simulink model "Test14Dof"  (R2024a)
settings: Solver=ode4  StartTime=0.0  StopTime=10.0  FixedStep=0.001  RelTol=1e-3
values from neighbouring files (symbols this model uses):
  EnvGrvty = 9.81    [Par.m]
  PlntBattChrgMax = 4.493    [Par.m]
  PlntBattNumCellSer = 96    [Par.m]
  PlntBattOpenCirctVolt = [3.17242 3.17242 3.17242 3.17242 3.17242 3.17242 3.17242;3.18272 3.18272 3.18272 3.18272 3.18272 3.18272 3.18272;3.19302 3.19302 3.19302 3.19302 3.19302 3.19302 3.19302;3.20331 3.20331 3.20331 3.20331 3.20331 3.20331 3.20331;3.21361 3.21361 3.21361 3.21361 3.21361 3.21361 3.21361;3.22391 3.22391 3.22391 3.22391 3.22391 3.22391 3.22391;3.23421 3.23421 3.23421 3.23421 3.23421 3.23421 3.23421;3.24451 ...(+5187 chars)    [Par.m]
  PlntBattSocInit = 0.6    [Par.m]
  PlntBattTempBpt = [-40 -30 -20 0 23 45 60]    [Par.m]
  PlntBattTempInitDegC = 25    [Par.m]
  PlntBattVoltSocBpt = [0 0.01 0.02 0.03 0.04 0.05 0.06 0.07 0.08 0.09 0.1 0.11 0.12 0.13 0.14 0.15 0.16 0.17 0.18 0.19 0.2 0.21 0.22 0.23 0.24 0.25 0.26 0.27 0.28 0.29 0.3 0.31 0.32 0.33 0.34 0.35 0.36 0.37 0.38 0.39 0.4 0.41 0.42 0.43 0.44 0.45 0.46 0.47 0.48 0.49 0.5 0.51 0.52 0.53 0.54 0.55 0.56 0.57 0.58 0.59 0.6 0.61 0.62 0.63 0.64 0.65 0.66 0.67 0.68 0.69 0.7 0.71 0.72 0.73 0.74 0.75 0.76 0.77 0.78 0.79 0.8 0.81  ...(+91 chars)    [Par.m]
  PlntDCDCVoltInit = 650    [Par.m]
  PlntDriveshftDamp = 100    [Par.m]
  PlntDriveshftStiff = 500    [Par.m]
  PlntEM1RotDamp = 0.001    [Par.m]
  PlntEM1RotInertia = 0.01    [Par.m]
  PlntEM2RotDamp = 0.001    [Par.m]
  PlntEM2RotInertia = 0.01    [Par.m]
  PlntEM3RotDamp = 0.001    [Par.m]
  PlntEM3RotInertia = 0.01    [Par.m]
  PlntEM4RotDamp = 0.001    [Par.m]
  PlntEM4RotInertia = 0.01    [Par.m]
  PlntEMWhlGearRatioFL = 11.04    [Par.m]
  PlntEMWhlGearRatioFR = 11.04    [Par.m]
  PlntEMWhlGearRatioRL = 11.04    [Par.m]
  PlntEMWhlGearRatioRR = 11.04    [Par.m]
  PlntSteerGearRatio = 52.025    [Par.m]
  PlntVehCGHgtAxl = 0.375    [Par.m]
  PlntVehDstCGFrntAxl = 1.61    [Par.m]
  PlntVehDstCGRearAxl = 1.39    [Par.m]
  PlntVehFrntUnsprgMass = 100    [Par.m]
  PlntVehInitLatPos = 0    [Par.m]
  PlntVehInitLatVel = 0    [Par.m]
  PlntVehInitLongPos = 0    [Par.m]
  PlntVehInitLongVel = 0    [Par.m]
  PlntVehInitPitchAng = 0    [Par.m]
  PlntVehInitPitchRate = 0    [Par.m]
  PlntVehInitRollAng = 0    [Par.m]
  PlntVehInitRollRate = 0    [Par.m]
  PlntVehInitVertPos = 0    [Par.m]
  PlntVehInitVertVel = 0    [Par.m]
  PlntVehInitYawAng = 0    [Par.m]
  PlntVehInitYawRate = 0    [Par.m]
  PlntVehMass = 2497    [Par.m]
  PlntVehPitchMomentInertia = 1922.7    [Par.m]
  PlntVehRearUnsprgMass = 100    [Par.m]
  PlntVehRollMomentInertia = 432.33333333333331    (= 432.333333333)    [Par.m]
  PlntVehTrckWdth = [1.685,1.685]    [Par.m]
  PlntVehYawMomentInertia = 2066    [Par.m]
  PlntWhlNumFrnt = 2    [Par.m]
  PlntWhlNumRear = 2    [Par.m]
  PlntWhlPrsFrnt = 220000    [Par.m]
  PlntWhlPrsRear = 220000    [Par.m]
undefined symbols (not defined in the file or in its folder): BdyFrm, InertFrm, PlntTrnsfrCaseAxlSpdLock, PlntTrnsfrCaseTrqSplitRatio
libraries: autolibsharedcoupling x12, autolibsharedcommon x12, autolibutils x10, autolibmappedmotor x4, autolibcoupling x4, matrix_library x4, vehdynlibsuspension x2, vehdynlibtire x2, vehdynlibtirecommon x2, vehdynlibsteering x2, shared6dof x2, autolibdatasheetbattery x1
(part 4 of 7)

== system Test14Dof/Subsystem/Vehicle 14 DoF model/Front Suspension/Wheel2SuspFrntOnly ==
  Veh : Inport
  Wheels : Inport  Port=2
  SuspWheel : Inport  Port=3
  Bus Creator : BusCreator  Inputs=2
  Bus Creator1 : BusCreator  Inputs=2
  Bus Selector : BusSelector  OutputSignals=Fext,WhlAng
  Bus Selector7 : BusSelector  OutputSignals=Omega,Fx,Fy,Mx,My,Mz,Re,z,zdot,Kappa,Alpha
  Constant : Constant  Value=repmat(eye(3),[1,1,PlntWhlNumFrnt])
  Math Function : Math  Operator=transpose  SignedPower=on
  Math Function1 : Math  Operator=transpose  SignedPower=on
  Reshape3 : Reshape
  Reshape4 : Reshape
  Selector2 : Selector  NumberOfDimensions=2  InputPortWidth=3  IndexOptions=Index vector (dialog),Select all  Indices=3,1  OutputSizes=1,1
  Selector3 : Selector  NumberOfDimensions=2  InputPortWidth=3  IndexOptions=Index vector (dialog),Select all  Indices=1,1  OutputSizes=1,1
  Signal Specification : SignalSpecification  Dimensions=PlntWhlNumFrnt
  Signal Specification1 : SignalSpecification  Dimensions=PlntWhlNumFrnt
  Signal Specification2 : SignalSpecification  Dimensions=PlntWhlNumFrnt
  Suspension Routing : Subsystem
  Vector Concatenate1 : Concatenate  NumInputs=3  Mode=Multidimensional array  ConcatenateDimension=2
  Vector Concatenate8 : Concatenate  NumInputs=3  Mode=Multidimensional array  ConcatenateDimension=2
  Wheel to Body Transform : Subsystem
  Wheels2Susp : Outport  VectorParamsAs1DForOutWhenUnconnected=off
  wires:
  Signal Specification1/1 -> Vector Concatenate8/2
  Signal Specification/1 -> Vector Concatenate8/1
  Veh/1 -> Suspension Routing/13(Veh)
  Bus Creator/1 -> Bus Creator1/2  "Steering"
  Reshape3/1 -> Bus Creator/2  "WhlCmb"
  Suspension Routing/1(SuspFrame) -> Bus Creator1/1  "SuspFrame"
  Bus Creator1/1 -> Wheels2Susp/1
  Reshape4/1 -> Bus Creator/1  "WhlAng"
  Wheel to Body Transform/3(Fz) -> Suspension Routing/4(Fz)  "Fz"
  Bus Selector/2 -> [WheelAngles], Wheel to Body Transform/4(WheelAngles)  "<WhlAng>"
  Wheels/1 -> Bus Selector7/1
  Math Function/1 -> Wheel to Body Transform/1(Forces)
  Vector Concatenate8/1 -> Math Function/1
  Wheel to Body Transform/1(Fx) -> Suspension Routing/2(Fx)  "Fx"
  Wheel to Body Transform/2(Fy) -> Suspension Routing/3(Fy)  "Fy"
  SuspWheel/1 -> Bus Selector/1
  Bus Selector/1 -> Signal Specification2/1  "<Fext>"
  Signal Specification2/1 -> Vector Concatenate8/3
  Selector2/1 -> Reshape4/1
  [WheelAngles] -> Selector2/1, Selector3/1
  Selector3/1 -> Reshape3/1
  Wheel to Body Transform/4(Mx) -> Suspension Routing/5(<Mx>)
  Wheel to Body Transform/5(My) -> Suspension Routing/6(<My>)
  Wheel to Body Transform/6(Mz) -> Suspension Routing/7(<Mz>)
  Vector Concatenate1/1 -> Math Function1/1
  Math Function1/1 -> Wheel to Body Transform/2(Moments)
  Constant/1 -> Wheel to Body Transform/3(DCM)
  Bus Selector7/1 -> Suspension Routing/1(Omega)  "<Omega>"
  Bus Selector7/2 -> Signal Specification/1  "<Fx>"
  Bus Selector7/3 -> Signal Specification1/1  "<Fy>"
  Bus Selector7/4 -> Vector Concatenate1/1  "<Mx>"
  Bus Selector7/5 -> Vector Concatenate1/2  "<My>"
  Bus Selector7/6 -> Vector Concatenate1/3  "<Mz>"
  Bus Selector7/7 -> Wheel to Body Transform/5(Re), Suspension Routing/8(<Re>)  "<Re>"
  Bus Selector7/8 -> Suspension Routing/9(<z>)  "<z>"
  Bus Selector7/9 -> Suspension Routing/10(<zdot>)  "<zdot>"
  Bus Selector7/10 -> Suspension Routing/11(<Kappa>)  "<Kappa>"
  Bus Selector7/11 -> Suspension Routing/12(<Alpha>)  "<Alpha>"

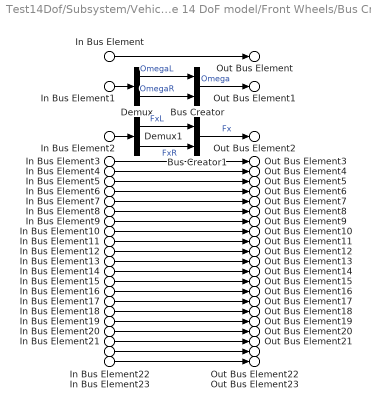
== system Test14Dof/Subsystem/Vehicle 14 DoF model/Front Wheels/Bus Creator ==
  In Bus Element : Inport  PortName=Info  Element=AxlTrq
  In Bus Element1 : Inport  PortName=Info  Element=Omega
  In Bus Element2 : Inport  PortName=Info  Element=Fx
  In Bus Element3 : Inport  PortName=Info  Element=Fy
  In Bus Element4 : Inport  PortName=Info  Element=Fz
  In Bus Element5 : Inport  PortName=Info  Element=Mx
  In Bus Element6 : Inport  PortName=Info  Element=My
  In Bus Element7 : Inport  PortName=Info  Element=Mz
  In Bus Element8 : Inport  PortName=Info  Element=Vx
  In Bus Element9 : Inport  PortName=Info  Element=Vy
  In Bus Element10 : Inport  PortName=Info  Element=Re
  In Bus Element11 : Inport  PortName=Info  Element=Kappa
  In Bus Element12 : Inport  PortName=Info  Element=Alpha
  In Bus Element13 : Inport  PortName=Info  Element=a
  In Bus Element14 : Inport  PortName=Info  Element=b
  In Bus Element15 : Inport  PortName=Info  Element=Gamma
  In Bus Element16 : Inport  PortName=Info  Element=psidot
  In Bus Element17 : Inport  PortName=Info  Element=BrkTrq
  In Bus Element18 : Inport  PortName=Info  Element=BrkPrs
  In Bus Element19 : Inport  PortName=Info  Element=z
  In Bus Element20 : Inport  PortName=Info  Element=zdot
  In Bus Element21 : Inport  PortName=Info  Element=Gnd
  In Bus Element22 : Inport  PortName=Info  Element=GndFz
  In Bus Element23 : Inport  PortName=Info  Element=Prs
  Bus Creator : BusCreator  Inputs=2
  Bus Creator1 : BusCreator  Inputs=2
  Demux : Demux  Outputs=2
  Demux1 : Demux  Outputs=2
  Out Bus Element : Outport  PortName=Wheels  Element=AxlTrq
  Out Bus Element1 : Outport  PortName=Wheels  Element=Omega
  Out Bus Element2 : Outport  PortName=Wheels  Element=Fx
  Out Bus Element3 : Outport  PortName=Wheels  Element=Fy
  Out Bus Element4 : Outport  PortName=Wheels  Element=Fz
  Out Bus Element5 : Outport  PortName=Wheels  Element=Mx
  Out Bus Element6 : Outport  PortName=Wheels  Element=My
  Out Bus Element7 : Outport  PortName=Wheels  Element=Mz
  Out Bus Element8 : Outport  PortName=Wheels  Element=Vx
  Out Bus Element9 : Outport  PortName=Wheels  Element=Vy
  Out Bus Element10 : Outport  PortName=Wheels  Element=Re
  Out Bus Element11 : Outport  PortName=Wheels  Element=Kappa
  Out Bus Element12 : Outport  PortName=Wheels  Element=Alpha
  Out Bus Element13 : Outport  PortName=Wheels  Element=a
  Out Bus Element14 : Outport  PortName=Wheels  Element=b
  Out Bus Element15 : Outport  PortName=Wheels  Element=Gamma
  Out Bus Element16 : Outport  PortName=Wheels  Element=psidot
  Out Bus Element17 : Outport  PortName=Wheels  Element=BrkTrq
  Out Bus Element18 : Outport  PortName=Wheels  Element=BrkPrs
  Out Bus Element19 : Outport  PortName=Wheels  Element=z
  Out Bus Element20 : Outport  PortName=Wheels  Element=zdot
  Out Bus Element21 : Outport  PortName=Wheels  Element=Gnd
  Out Bus Element22 : Outport  PortName=Wheels  Element=GndFz
  Out Bus Element23 : Outport  PortName=Wheels  Element=Prs
  wires:
  In Bus Element16/1 -> Out Bus Element16/1
  In Bus Element10/1 -> Out Bus Element10/1
  In Bus Element3/1 -> Out Bus Element3/1
  In Bus Element18/1 -> Out Bus Element18/1
  In Bus Element12/1 -> Out Bus Element12/1
  In Bus Element11/1 -> Out Bus Element11/1
  In Bus Element20/1 -> Out Bus Element20/1
  In Bus Element13/1 -> Out Bus Element13/1
  In Bus Element8/1 -> Out Bus Element8/1
  In Bus Element14/1 -> Out Bus Element14/1
  In Bus Element15/1 -> Out Bus Element15/1
  In Bus Element17/1 -> Out Bus Element17/1
  In Bus Element19/1 -> Out Bus Element19/1
  In Bus Element22/1 -> Out Bus Element22/1
  In Bus Element21/1 -> Out Bus Element21/1
  In Bus Element23/1 -> Out Bus Element23/1
  In Bus Element1/1 -> Demux/1
  In Bus Element/1 -> Out Bus Element/1
  In Bus Element4/1 -> Out Bus Element4/1
  In Bus Element6/1 -> Out Bus Element6/1
  In Bus Element5/1 -> Out Bus Element5/1
  In Bus Element9/1 -> Out Bus Element9/1
  In Bus Element7/1 -> Out Bus Element7/1
  Demux/1 -> Bus Creator/1  "OmegaL"
  Demux/2 -> Bus Creator/2  "OmegaR"
  Bus Creator/1 -> Out Bus Element1/1  "Omega"
  Bus Creator1/1 -> Out Bus Element2/1  "Fx"
  Demux1/2 -> Bus Creator1/2  "FxR"
  Demux1/1 -> Bus Creator1/1  "FxL"
  In Bus Element2/1 -> Demux1/1

== system Test14Dof/Subsystem/Vehicle 14 DoF model/Front Wheels/Front Friction ==
  u : Inport
  Selector1 : Selector  InputPortWidth=4  IndexOptions=Index vector (dialog)  Indices=[1 2]  OutputSizes=1
  y : Outport
  wires:
  Selector1/1 -> y/1
  u/1 -> Selector1/1

== system Test14Dof/Subsystem/Vehicle 14 DoF model/Front Wheels/Front Ground ==
  u : Inport
  Selector1 : Selector  InputPortWidth=4  IndexOptions=Index vector (dialog)  Indices=[1 2]  OutputSizes=1
  y : Outport
  wires:
  u/1 -> Selector1/1
  Selector1/1 -> y/1

== system Test14Dof/Subsystem/Vehicle 14 DoF model/Front Wheels/MF Tires Vector ==
  BrkPrs : Inport
  AxlTrq : Inport  Port=2
  Vx : Inport  Port=3
  Vy : Inport  Port=4
  Camber : Inport  Port=5
  YawRate : Inport  Port=6
  Fext : Inport  Port=7
  Prs : Inport  Port=8  Unit=Pa
  ScaleFctrs : Inport  Port=9  Unit=1
  Gnd : Inport  Port=10
  Combined Slip Wheel 2DOF1 : vehdynlibtire/Combined Slip Wheel 2DOF  tireType=SUV 265/50R20  BrakeType=Disc  vertType=Magic Formula  plySteer=off  turnslip=on  mu_static=.3  mu_kinetic=.2  disk_abore=.05  Rm=.177  num_pads=2  drum_abore=0.0508  drum_a=0.123  drum_c=0.212  drum_r=0.15  drum_theta1=0  drum_theta2=126  brake_p_bpt=[1 11.4736842105263 21.9473684210526 32.4210526315789 42.8947368421053 53.3684210526316 63.8421052631579 74.3157894736842 84.7894736842105 95.2631578947368 105.736842105263 116.210526315789 126.684210526316 137.157894736842 147.631578947368 158.105263157895 168.578947368421 179.052631578947 189.526315789474 200]  brake_n_bpt=[0 52.6315789473684 105.263157894737 157.894736842105 210.526315789474 263.157894736842 315.789473684211 368.421052631579 421.052631578947 473.684210526316 526.315789473684 578.947368421053 631.578947368421 684.210526315789 736.842105263158 789.473684210526 842.105263157895 894.736842105263 947.368421052632 1000]  f_brake_t=[43.4900602404453 42.5056030554862 41.5350898940194 40.5780454442085 39.6340111501808 38.7025443887544 37.7832176914519 36.8756180088306 35.9793460143796 35.0940154454303 34.2192524787115 33.3546951383474 32.4999927342521 31.6548053290159 30.8188032315107 29.991666515561 29.1730845621415 28.362755623661 27.5603864089927 26.765691687993;498.991217495636 487.695866636631 476.560505099801 465.579679307235 454.748127933653 444.060772460445 433.51270824929 423.099196101319 412.81565427025 402.657650900201 392.620896861006 382.701238955775 372.894653477208 363.197240090814 353.605216024701 344.114910546964 334.722759712992 325.425301366216 316.219170376863 307.10109410434;954.492374750826 932.886130217776 911.585920305583 890.581313170261 869.862244717126 849.419000532136 829.242198807128 809.322774193808 789.651962526121 770.221286354971 751.0225412433 732.047782773203 713.289314220164 694.739674852612 676.391628817892 658.238154578366 640.272434863842 622.48784710877 604.877954344734 587.436496520688;1409.99353200602 1378.07639379892 1346.61133551136 1315.58294703329 1284.9763615006 1254.77722860383 1224.97168936497 1195.5463522863 1166.48827078199 1137.78492180974 1109.42418562559 1081.39432659063 1053.68397496312 1026.28210961441 999.178041611083 972.361398609768 945.822110014692 919.550392851325 893.536738312604 867.771898937035;1865.49468926121 1823.26665738007 1781.63675071715 1740.58458089631 1700.09047828407 1660.13545667552 1620.7011799228 1581.76993037878 1543.32457903786 1505.34855726451 1467.82583000789 1430.74087040806 1394.07863570608 1357.82454437621 1321.96445440427 1286.48464264117 1251.37178516554 1216.61293859388 1182.19552228048 1148.10730135338;2320.9958465164 2268.45692096121 2216.66216592293 2165.58621475934 2115.20459506754 2065.49368474721 2016.43067048064 1967.99350847127 1920.16088729373 1872.91219271928 1826.22747439018 1780.08741422549 1734.47329644903 1689.36697913801 1644.75086719747 1600.60788667257 1556.92146031639 1513.67548433643 1470.85430624835 1428.44270376973;2776.49700377159 2713.64718454235 2651.68758112871 2590.58784862237 2530.31871185102 2470.8519128189 2412.16016103848 2354.21708656376 2296.9971955496 2240.47582817405 2184.62911877248 2129.43395804292 2074.86795719199 2020.9094138998 1967.53727999066 1914.73113070398 1862.47113546724 1810.73803007899 1759.51309021622 1708.77810618608;3231.99816102678 3158.8374481235 3086.71299633449 3015.58948248539 2945.43282863449 2876.21014089059 2807.88965159632 2740.44066465625 2673.83350380547 2608.03946362882 2543.03076315477 2478.78050186034 2415.26261793494 2352.4518486616 2290.32369278385 2228.85437473538 2168.02081061809 2107.80057582154 2048.17187418409 1989.11350860242;3687.49931828197 3604.02771170464 3521.73841154027 3440.59111634842 3360.54694541796 3281.56836896228 3203.61914215416 3126.66424274874 3050.66981206134 2975.60309908359 2901.43240753707 2828.12704567777 2755.6572786779 2683.9942834234 2613.11010557704 2542.97761876678 2473.57048576894 2404.8631215641 2336.83065815196 2269.44891101877;4143.00047553716 4049.21797528579 3956.76382674606 3865.59275021144 3775.66106220143 3686.92659703397 3599.34863271199 3512.88782084123 3427.50612031721 3343.16673453836 3259.83405191936 3177.4735894952 3096.05193942085 3015.5367181852 2935.89651837023 2857.10086279818 2779.12016091979 2701.92566730665 2625.48944211983 2549.78431343512;4598.50163279235 4494.40823886693 4391.78924195184 4290.59438407447 4190.77517898491 4092.28482510566 3995.07812326983 3899.11139893372 3804.34242857308 3710.73036999313 3618.23569630166 3526.82013331263 3436.44660016381 3347.079152947 3258.68293116342 3171.22410682959 3084.66983607064 2998.98821304921 2914.1482260877 2830.11971585147;5054.00279004754 4939.59850244808 4826.81465715762 4715.59601793749 4605.88929576838 4497.64305317735 4390.80761382767 4285.3349770262 4181.17873682896 4078.2940054479 3976.63734068395 3876.16667713006 3776.84126090677 3678.62158770879 3581.46934395661 3485.34735086099 ...(+2764 chars)]  tireParamSet=vdynPassCar.mat  PRESMAX=1000000  PRESMIN=10000  FZMAX=12400  FZMIN=100  VXLOW=0.1  KPUMAX=1.5  KPUMIN=-1.5  ALPMAX=1.5  ALPMIN=-1.5  CAMMAX=0.17453  CAMMIN=-0.17453  LONGVL=16.7  FxRelFreqLwrLim=200*pi  FyRelFreqLwrLim=200*pi  MyRelFreqLwrLim=100*pi  omegao=0  br=1e-3  UNLOADED_RADIUS=0.3869  NOMPRES=269000  FNOMIN=6200  WIDTH=0.265  RIM_RADIUS=0.254  MASS=16.15  IYY=2.081  GRAVITY=-9.81  zo=0  zdoto=0  BREFF=8.25094594147963  DREFF=0.260468730454265  FREFF=0.0735298544471851  Q_RE0=1.00866439868088  Q_V1=0.000760413786224011  Q_V2=0.0463384792019201  Q_FZ1=0  Q_FZ2=15.6870832810226  Q_FZ3=0  Q_FCX=0.138643970247602  Q_FCY=0.10843499565426  Q_FCY2=-0.465763352339538  PFZ1=0.69958166705601  VERTICAL_STIFFNESS=207885.061134007  VERTICAL_DAMPING=500  BOTTOM_OFFST=.01  BOTTOM_STIFF=2e6  LONGITUDINAL_STIFFNESS=388714.175879854  LATERAL_STIFFNESS=157087.404633332  PCFX1=0.18539229191199  PCFX2=0  PCFX3=0  PCFY1=0.163183345037677  PCFY2=0  PCFY3=0.249094918231954  Q_RA1=0.675942571700787  Q_RA2=0.73800463546164  Q_RB1=1.04487486456705  Q_RB2=-1.191763806629  PCX1=1.58523057950359  PDX1=1.0239116238178  PDX2=-0.0842405110022724  PDX3=0  PEX1=0.110312777158455  PEX2=0.313468516038146  PEX3=0  PEX4=0.0016060905760045  PKX1=21.3872544684023  PKX2=14.0006541873175  PKX3=-0.405326109653452  PHX1=0.000212599305364818  PHX2=0.00115950515263055  PVX1=1.59236164471432e-05  PVX2=0.000104321112127671  PPX1=-0.349461321276586  PPX2=0.387840040616429  PPX3=-0.0969947336569324  PPX4=0.0632271859795801  RBX1=12.7633329850276  RBX2=9.5787123658471  RBX3=0  RCX1=1.02796280922059  REX1=-0.45202516851367  REX2=-0.47304886171176  RHX1=0.000233272373115809  QSX1=-0.00788307788961443  QSX2=0.954629515459396  QSX3=0.0155855777667025  QSX4=0.125904607142414  QSX5=1.01110069703963  QSX6=20.1938577118433  QSX7=0.310818120717083  QSX8=-0.0430823751139655  QSX9=0.636494404888216  QSX10=0.142438060591663  QSX11=0.346766530036373  QSX12=0  QSX13=0  QSX14=0  PPMX1=0  PCY1=1.34299950037631  PDY1=0.878267729082195  PDY2=-0.0644597923147385  PDY3=0  PEY1=-0.809776534470972  PEY2=-0.600180598867198  PEY3=0.0991732552633487  PEY4=-6.5577974035573  PEY5=0  PKY1=-15.5714726518315  PKY2=1.73126522291751  PKY3=0.365349873517229  PKY4=1.98176755955416  PKY5=0  PKY6=-0.884005199550313  PKY7=-0.237259727611847  PHY1=-0.00183370557235628  PHY2=0.00346401302716671  PVY1=-0.00675427560163264  PVY2=0.036379218103843  PVY3=-0.163543984089166  PVY4=-0.491003349625726  PPY1=-0.62059646553185  PPY2=-0.0647824842338686  PPY3=-0.164648843290686  PPY4=0.283193909060098  PPY5=0  RBY1=10.7588809173639  RBY2=7.70420065295029  RBY3=3.40283755070691e-06  RBY4=0  RCY1=1.06691874059059  REY1=0.308244924574305  REY2=7.48775032604508e-06  RHY1=0.0118479204960415  RHY2=7.63650177161071e-06  RVY1=0.0560024425050078  RVY2=7.48487127056197e-06  RVY3=0  RVY4=98.4047026517149  RVY5=2.02759273900054  RVY6=15.7623064923347  QSY1=0.00699077564863536  QSY2=0  QSY3=0.00153535478298811  QSY4=8.55710322455322e-05  QSY5=0  QSY6=0  QSY7=0.89443879773793  QSY8=-0.403227641260894  QBZ1=11.666656027484  QBZ2=-1.30355438574485  QBZ3=0  QBZ4=0.177918305399071  QBZ5=-0.162481135068033  QBZ6=0  QBZ9=30.1445534682089  QBZ10=0  QCZ1=1.29026978207574  QDZ1=0.0886972644991399  QDZ2=-0.0058634820161856  QDZ3=0.3805597481383  QDZ4=0  QDZ6=0.00160914918118959  QDZ7=-0.00211036330862154  QDZ8=-0.13921904912557  QDZ9=0.00816585550028243  QDZ10=0  QDZ11=0  QEZ1=-2.19802254534746  QEZ2=1.01850535789165  QEZ3=0  QEZ4=0.278379679112054  QEZ5=-0.548414722765386  QHZ1=0.00148361198869669  QHZ2=0.00202017567585904  QHZ3=0.240316641332066  QHZ4=-0.210114035738085  PPZ1=-0.443927982388615  PPZ2=0  SSZ1=0.00914999585397887  SSZ2=0.0389830656052735  SSZ3=0  SSZ4=0  PDXP1=0.396718274678791  PDXP2=0  PDXP3=0  PKYP1=1.00587060633573  PDYP1=0.40483048923438  PDYP2=0  PDYP3=0  PDYP4=0  PHYP1=0.992731942067188  PHYP2=0.150352945499914  PHYP3=0  PHYP4=-3.98988682633674  PECP1=0.502379254513503  PECP2=0  QDTP1=10.0178654287947  QCRP1=0.200627747200702  QCRP2=0.0995735881599772  QBRP1=0.0997107127960717  QDRP1=1.01432910167423  QDRP2=0  aMode=2
  Terminator{7..13} (7 alike) : Terminator
  Wheels : Outport  VectorParamsAs1DForOutWhenUnconnected=off
  wires:
  Vy/1 -> Combined Slip Wheel 2DOF1/4
  Combined Slip Wheel 2DOF1/8 -> Terminator13/1
  Combined Slip Wheel 2DOF1/7 -> Terminator12/1
  Combined Slip Wheel 2DOF1/6 -> Terminator11/1
  Combined Slip Wheel 2DOF1/5 -> Terminator10/1
  Combined Slip Wheel 2DOF1/4 -> Terminator9/1
  Combined Slip Wheel 2DOF1/3 -> Terminator8/1
  Combined Slip Wheel 2DOF1/2 -> Terminator7/1
  Fext/1 -> Combined Slip Wheel 2DOF1/9
  Gnd/1 -> Combined Slip Wheel 2DOF1/8
  Prs/1 -> Combined Slip Wheel 2DOF1/7
  YawRate/1 -> Combined Slip Wheel 2DOF1/6
  Camber/1 -> Combined Slip Wheel 2DOF1/5
  Vx/1 -> Combined Slip Wheel 2DOF1/3
  AxlTrq/1 -> Combined Slip Wheel 2DOF1/2
  BrkPrs/1 -> Combined Slip Wheel 2DOF1/1
  Combined Slip Wheel 2DOF1/1 -> Wheels/1
  ScaleFctrs/1 -> Combined Slip Wheel 2DOF1/10

== system Test14Dof/Subsystem/Vehicle 14 DoF model/Front Wheels/Subsystem ==
  lamda_mu_x : Inport
  lamda_mu_y : Inport  Port=2
  Front Pressure : vehdynlibtirecommon/Constant  const=PlntWhlPrsFrnt  numWheels=PlntWhlNumFrnt
  scale factors with friction : Subsystem  mask{numWheels=PlntWhlNumFrnt}
      mask prompts: numWheels "Number of wheels"
  Prs : Outport
  ScaleFctrs : Outport  Port=2
  wires:
  lamda_mu_y/1 -> scale factors with friction/2(lamda_mu_y)
  scale factors with friction/1(lambdas) -> ScaleFctrs/1
  lamda_mu_x/1 -> scale factors with friction/1(lamda_mu_x)
  Front Pressure/1 -> Prs/1

== system Test14Dof/Subsystem/Vehicle 14 DoF model/Rear Axle/Rear Axle ==
  Prs1 : Inport
  Prs2 : Inport  Port=2
  DriveshftTrq : Inport  Port=3
  Axl1Trq : Inport  Port=4
  Axl2Trq : Inport  Port=5
  Bus Creator : BusCreator  Inputs=2
  Bus Creator1 : BusCreator  Inputs=2
  Bus Selector : BusSelector  OutputSignals=DriveshftTrq3
  Bus Selector1 : BusSelector  OutputSignals=DriveshftTrq4
  Gearbox_RL : autolibcoupling/Gearbox  port_config=Simulink  input_config=Torque input - velocity output  DiffEffModelPopup=Constant  InterpMethod=Flat  dirSwitch=on  extTamb=off  N=PlntEMWhlGearRatioRL  J1=PlntEMWhlGearInInertiaRL  J2=PlntEMWhlGearOutInertiaRL  b1=PlntEMWhlGearInDampRL  b2=PlntEMWhlGearOutDampRL  theta1_o=0  w1_o=PlntEMWhlGearInInitVelRL  eta=PlntEMWhlGearEffRL  eta_tbl=reshape([0.64 0.76 0.8 0.81 0.83 0.84 0.84 0.56 0.73 0.78 0.8 0.83 0.84 0.84 0.54 0.71 0.77 0.8 0.82 0.84 0.84 0.53 0.71 0.77 0.8 0.83 0.84 0.84 0.51 0.71 0.77 0.8 0.83 0.84 0.85 0.52 0.7 0.77 0.8 0.83 0.84 0.85 0.51 0.71 0.76 0.79 0.83 0.84 0.85 0.5 0.69 0.76 0.79 0.82 0.84 0.85 0.45 0.68 0.75 0.78 0.82 0.84 0.85 0.43 0.67 0.74 0.78 0.81 0.83 0.84 0.38 0.63 0.71 0.75 0.8 0.82 0.83 0.81 0.86 0.88 0.89 0.89 0.89 0.9 0.77 0.85 0.87 0.88 0.89 0.9 0.9 0.72 0.82 0.86 0.87 0.88 0.89 0.9 0.68 0.8 0.84 0.86 0.88 0.89 0.89 0.67 0.8 0.84 0.86 0.88 0.89 0.9 0.67 0.8 0.84 0.86 0.88 0.89 0.9 0.65 0.8 0.84 0.86 0.88 0.89 0.9 0.64 0.79 0.83 0.86 0.88 0.89 0.9 0.63 0.78 0.83 0.86 0.88 0.89 0.9 0.59 0.76 0.82 0.85 0.87 0.89 0.9 0.53 0.73 0.8 0.83 0.86 0.88 0.89], 7, 11, 2)  Trq_bpts=[25, 50, 75, 100, 150, 200, 250]  omega_bpts=[52.4 78.5 105 131 157 183 209 262 314 419 524]  Temp_bpts=[290 358]  Tamb=297.15  blkID=0
  Gearbox_RR : autolibcoupling/Gearbox  port_config=Simulink  input_config=Torque input - velocity output  DiffEffModelPopup=Constant  InterpMethod=Flat  dirSwitch=on  extTamb=off  N=PlntEMWhlGearRatioRR  J1=PlntEMWhlGearInInertiaRR  J2=PlntEMWhlGearOutInertiaRR  b1=PlntEMWhlGearInDampRR  b2=PlntEMWhlGearOutDampRR  theta1_o=0  w1_o=PlntEMWhlGearInInitVelRR  eta=PlntEMWhlGearEffRR  eta_tbl=reshape([0.64 0.76 0.8 0.81 0.83 0.84 0.84 0.56 0.73 0.78 0.8 0.83 0.84 0.84 0.54 0.71 0.77 0.8 0.82 0.84 0.84 0.53 0.71 0.77 0.8 0.83 0.84 0.84 0.51 0.71 0.77 0.8 0.83 0.84 0.85 0.52 0.7 0.77 0.8 0.83 0.84 0.85 0.51 0.71 0.76 0.79 0.83 0.84 0.85 0.5 0.69 0.76 0.79 0.82 0.84 0.85 0.45 0.68 0.75 0.78 0.82 0.84 0.85 0.43 0.67 0.74 0.78 0.81 0.83 0.84 0.38 0.63 0.71 0.75 0.8 0.82 0.83 0.81 0.86 0.88 0.89 0.89 0.89 0.9 0.77 0.85 0.87 0.88 0.89 0.9 0.9 0.72 0.82 0.86 0.87 0.88 0.89 0.9 0.68 0.8 0.84 0.86 0.88 0.89 0.89 0.67 0.8 0.84 0.86 0.88 0.89 0.9 0.67 0.8 0.84 0.86 0.88 0.89 0.9 0.65 0.8 0.84 0.86 0.88 0.89 0.9 0.64 0.79 0.83 0.86 0.88 0.89 0.9 0.63 0.78 0.83 0.86 0.88 0.89 0.9 0.59 0.76 0.82 0.85 0.87 0.89 0.9 0.53 0.73 0.8 0.83 0.86 0.88 0.89], 7, 11, 2)  Trq_bpts=[25, 50, 75, 100, 150, 200, 250]  omega_bpts=[52.4 78.5 105 131 157 183 209 262 314 419 524]  Temp_bpts=[290 358]  Tamb=297.15  blkID=0
  Info : Outport
  DriveshftSpd : Outport  Port=2
  Axl1Spd : Outport  Port=3
  Axl2Spd : Outport  Port=4
  wires:
  Gearbox_RL/2 -> Bus Creator1/1  "DriveshftSpd3"
  Gearbox_RR/1 -> Bus Creator/2  "Gearbox_RR_Info"
  Bus Selector/1 -> Gearbox_RL/1  "<DriveshftTrq3>"
  Bus Creator1/1 -> DriveshftSpd/1
  Bus Selector1/1 -> Gearbox_RR/1  "<DriveshftTrq4>"
  Bus Creator/1 -> Info/1
  Axl1Trq/1 -> Gearbox_RL/2
  Gearbox_RL/1 -> Bus Creator/1  "Gearbox_RL_Info"
  Axl2Trq/1 -> Gearbox_RR/2
  DriveshftTrq/1 -> Bus Selector1/1, Bus Selector/1
  Gearbox_RR/2 -> Bus Creator1/2  "DriveshftSpd4"
  Gearbox_RL/3 -> Axl1Spd/1
  Gearbox_RR/3 -> Axl2Spd/1

== system Test14Dof/Subsystem/Vehicle 14 DoF model/Rear Axle/Subsystem ==
  RSpdL : Inport
  RSpdR : Inport  Port=2
  OmegaL : Inport  Port=3
  OmegaR : Inport  Port=4
  Torsional Compliance4 : autolibsharedcoupling/Torsional Compliance  port_config=Simulink  extInfo=off  k=PlntDriveshftStiff  b=PlntDriveshftDamp  theta_o=PlntDriveshftInitDeflect  domega_o=PlntDriveshftInitVel  omega_c=PlntDriveshftDampCutoffFreq  blkID=0  aMode=6
  Torsional Compliance5 : autolibsharedcoupling/Torsional Compliance  port_config=Simulink  extInfo=off  k=PlntDriveshftStiff  b=PlntDriveshftDamp  theta_o=PlntDriveshftInitDeflect  domega_o=PlntDriveshftInitVel  omega_c=PlntDriveshftDampCutoffFreq  blkID=0  aMode=6
  RTrqL : Outport
  RTrqR : Outport  Port=2
  CTrqL : Outport  Port=3
  CTrqR : Outport  Port=4
  wires:
  RSpdR/1 -> Torsional Compliance5/1
  RSpdL/1 -> Torsional Compliance4/1
  Torsional Compliance5/2 -> CTrqR/1
  OmegaR/1 -> Torsional Compliance5/2
  Torsional Compliance4/1 -> RTrqL/1
  Torsional Compliance5/1 -> RTrqR/1
  Torsional Compliance4/2 -> CTrqL/1
  OmegaL/1 -> Torsional Compliance4/2

== system Test14Dof/Subsystem/Vehicle 14 DoF model/Rear Axle/Subsystem1 ==
  Omega : Inport
  Bus Selector : BusSelector  OutputSignals=OmegaL,OmegaR
  Omega_RL : Outport
  Omega_RR : Outport  Port=2
  wires:
  Bus Selector/2 -> Omega_RR/1  "<OmegaR>"
  Omega/1 -> Bus Selector/1
  Bus Selector/1 -> Omega_RL/1  "<OmegaL>"

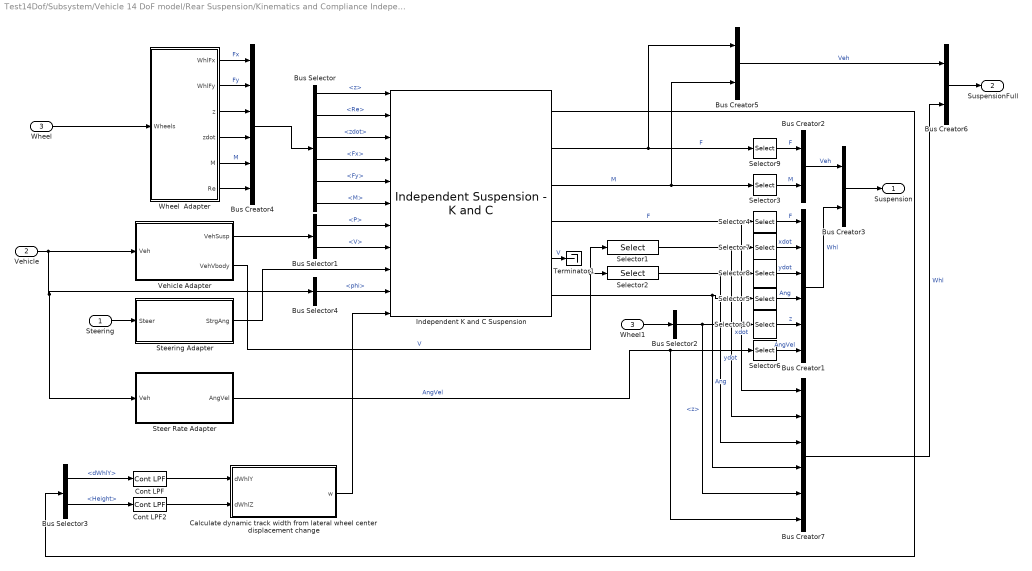
== system Test14Dof/Subsystem/Vehicle 14 DoF model/Rear Suspension/Kinematics and Compliance Independent Suspension ==
  Steering : Inport
  Vehicle : Inport  Port=2
  Wheel : Inport  Port=3
  Bus Creator1 : BusCreator  Inputs=6
  Bus Creator{2..3,5..6} (4 alike) : BusCreator  Inputs=2
  Bus Creator4 : BusCreator  Inputs=6
  Bus Creator7 : BusCreator  Inputs=6
  Bus Selector : BusSelector  OutputSignals=z,Re,zdot,Fx,Fy,M
  Bus Selector1 : BusSelector  OutputSignals=P,V
  Bus Selector2 : BusSelector  OutputSignals=SuspFrame.z
  Bus Selector3 : BusSelector  OutputSignals=dWhlY,Height
  Bus Selector4 : BusSelector  OutputSignals=InertFrm.Cg.Ang.phi
  Calculate dynamic track width from lateral wheel center displacement change : Subsystem  mask{w=PlntVehTrckWdth}
      mask prompts: w "vdynblks:vehdynVehBody6Dof:blkPrm_w"
      mask DialogControl w Prompt: Track widths [front, rear], w [m]:
  Cont LPF : autolibutils/Cont LPF  wc=100*2*pi  AbsoluteTolerance=auto  aMode=6
  Cont LPF2 : autolibutils/Cont LPF  wc=100*2*pi  AbsoluteTolerance=auto  aMode=6
  Independent K and C Suspension : vehdynlibsuspension/Independent Suspension - K and C  ActiveDampEn=off  NumAxl=2  NumWhlsByAxl=[2 2]  StrgEnByAxl=[1 0]  AntiSwayEnByAxl=[0 0]  WhlNumVec="[1  2  1  2]"  AxleNumVec="[1  1  2  2]"  SuspTypesByAxle="[1  1]"  SuspImage=suspkandc.png  IdealSuspEn=on  IdealSuspAxles="[1  2]"  tanTheta_FL=[0 0 0]  tanTheta_FR=[0 0 0]  tanTheta_RL=[0 0 0]  tanTheta_RR=[0 0 0]  SteerSign=1  LongitudinalSign=1  LateralSign=1  VerticalSign=1  WhlMzSign=1  tanTheta_SVSA_WC_FL=1  tanTheta_SVSA_WC_FR=1  tanTheta_SVSA_WC_RL=1  tanTheta_SVSA_WC_RR=1  tanTheta_SVSA_CP_FL=1  tanTheta_SVSA_CP_FR=1  tanTheta_SVSA_CP_RL=1  tanTheta_SVSA_CP_RR=1  SuspType=Independent front and rear  DrivetrainType=FWD  StrPlusDirection=Right  XPlusDirection=Front  YPlusDirection=Right  ZPlusDirection=Up  WhlMzDirection=Counter-clockwise  ShockType=Constant  ShckFrcVsCompRate=PlntSpKCShckFrcVsCompRate  MotRatios=PlntSpKCMotRatios  BumpSteer=PlntSpKCBumpSteer  BumpCamber=PlntSpKCBumpCamber  BumpCaster=PlntSpKCBumpCaster  LatWhlCtrDisp=PlntSpKCLatWhlCtrDisp  LngWhlCtrDisp=PlntSpKCLngWhlCtrDisp  NrmlWhlRates=PlntSpKCNrmlWhlRates  NrmlWhlFrcOff=PlntSpKCNrmlWhlFrcOff  RollSteer=[0 0 0 0]  RollCamber=[0 0 0 0]  RollCaster=[0 0 0 0]  RollStiffArb=PlntSpKCRollStiffArb  RollStiffNoArb=PlntSpKCRollStiffNoArb  RollStiffArbFrnt=800  RollStiffNoArbFrnt=0  RollStiffNoTwstRear=0  CambVsSteerAng=PlntSpKCCambVsSteerAng  CastVsSteerAng=PlntSpKCCastVsSteerAng  LngSteerCompl=PlntSpKCLngSteerCompl  LngCambCompl=PlntSpKCLngCambCompl  LngCastCompl=PlntSpKCLngCastCompl  LngWhlCtrCompl=PlntSpKCLngWhlCtrCompl  LatWhlCtrComplLngBrk=PlntSpKCLatWhlCtrComplLngBrk  LatSteerCompl=PlntSpKCLatSteerCompl  LatCambCompl=PlntSpKCLatCambCompl  LatWhlCtrComplLat=PlntSpKCLatWhlCtrComplLat  AlgnTrqSteerCompl=PlntSpKCAlgnTrqSteerCompl  AlgnTrqCambCompl=PlntSpKCAlgnTrqCambCompl  VrtLdTrnsfr=PlntSpKCVrtLdTrnsfr  StatToe=PlntSpKCStatToe  StatCamber=PlntSpKCStatCamber  StatCaster=PlntSpKCStatCaster  StatLdWhlR=PlntSpStatLdWhlR  MappedSuspEn=off  RollParamEn=off
  Selector1 : Selector  NumberOfDimensions=2  IndexOptions=Index vector (dialog),Select all  Indices=1,1  OutputSizes=1,1
  Selector10 : Selector  InputPortWidth=4  IndexOptions=Index vector (dialog)  Indices=[3 4]  OutputSizes=1
  Selector2 : Selector  NumberOfDimensions=2  IndexOptions=Index vector (dialog),Select all  Indices=2,1  OutputSizes=1,1
  Selector{3..6,9} (5 alike) : Selector  NumberOfDimensions=2  InputPortWidth=4  IndexOptions=Index vector (dialog),Index vector (dialog)  Indices=[1 2 3],[3 4]  OutputSizes=1,1
  Selector7 : Selector  InputPortWidth=4  IndexOptions=Index vector (dialog)  Indices=[3 4]  OutputSizes=1
  Selector8 : Selector  InputPortWidth=4  IndexOptions=Index vector (dialog)  Indices=[3 4]  OutputSizes=1
  Steer Rate Adapter : Subsystem
  Steering Adapter : Subsystem
  Terminator1 : Terminator
  Vehicle Adapter : Subsystem
  Wheel  Adapter : Subsystem
  Wheel1 : InportShadow  Port=3
  Suspension : Outport  VectorParamsAs1DForOutWhenUnconnected=off
  SuspensionFull : Outport  Port=2  VectorParamsAs1DForOutWhenUnconnected=off
  wires:
  Bus Creator3/1 -> Suspension/1
  Selector6/1 -> Bus Creator1/6  "AngVel"
  Bus Selector1/1 -> Independent K and C Suspension/7  "<P>"
  Independent K and C Suspension/4 -> Bus Creator7/1, Selector4/1  "F"
  Bus Creator4/1 -> Bus Selector/1
  Bus Selector/1 -> Independent K and C Suspension/1  "<z>"
  Independent K and C Suspension/6 -> Bus Creator7/4, Selector5/1  "Ang"
  Wheel1/1 -> Bus Selector2/1
  Bus Selector3/2 -> Cont LPF2/1  "<Height>"
  Calculate dynamic track width from lateral wheel center displacement change/1(w) -> Independent K and C Suspension/11
  Cont LPF/1 -> Calculate dynamic track width from lateral wheel center displacement change/1(dWhlY)
  Cont LPF2/1 -> Calculate dynamic track width from lateral wheel center displacement change/2(dWhlZ)
  Bus Selector2/1 -> Bus Creator7/5, Selector10/1  "<z>"
  Steering/1 -> Steering Adapter/1(Steer)
  Independent K and C Suspension/1 -> Bus Selector3/1
  Steering Adapter/1(StrgAng) -> Independent K and C Suspension/9
  Bus Creator1/1 -> Bus Creator3/2  "Whl"
  Wheel  Adapter/3(z) -> Bus Creator4/3
  Bus Selector/6 -> Independent K and C Suspension/6  "<M>"
  Bus Selector4/1 -> Independent K and C Suspension/10  "<phi>"
  Bus Selector/3 -> Independent K and C Suspension/3  "<zdot>"
  Wheel/1 -> Wheel  Adapter/1(Wheels)
  Bus Creator6/1 -> SuspensionFull/1
  Bus Creator7/1 -> Bus Creator6/2  "Whl"
  Bus Creator2/1 -> Bus Creator3/1  "Veh"
  Vehicle Adapter/2(VehVbody) -> Selector2/1, Selector1/1  "V"
  Selector2/1 -> Bus Creator7/3, Selector8/1  "ydot"
  Bus Selector1/2 -> Independent K and C Suspension/8  "<V>"
  Selector5/1 -> Bus Creator1/4  "Ang"
  Selector7/1 -> Bus Creator1/2  "xdot"
  Selector8/1 -> Bus Creator1/3  "ydot"
  Vehicle/1 -> Steer Rate Adapter/1(Veh), Bus Selector4/1, Vehicle Adapter/1(Veh)
  Bus Selector/5 -> Independent K and C Suspension/5  "<Fy>"
  Wheel  Adapter/2(WhlFy) -> Bus Creator4/2  "Fy"
  Independent K and C Suspension/5 -> Terminator1/1  "V"
  Selector3/1 -> Bus Creator2/2  "M"
  Wheel  Adapter/1(WhlFx) -> Bus Creator4/1  "Fx"
  Wheel  Adapter/4(zdot) -> Bus Creator4/4
  Independent K and C Suspension/3 -> Bus Creator5/2, Selector3/1  "M"
  Selector10/1 -> Bus Creator1/5  "z"
  Independent K and C Suspension/2 -> Bus Creator5/1, Selector9/1  "F"
  Bus Creator5/1 -> Bus Creator6/1  "Veh"
  Wheel  Adapter/5(M) -> Bus Creator4/5  "M"
  Steer Rate Adapter/1(AngVel) -> Bus Creator7/6, Selector6/1  "AngVel"
  Bus Selector/4 -> Independent K and C Suspension/4  "<Fx>"
  Wheel  Adapter/6(Re) -> Bus Creator4/6
  Selector1/1 -> Bus Creator7/2, Selector7/1  "xdot"
  Bus Selector3/1 -> Cont LPF/1  "<dWhlY>"
  Selector9/1 -> Bus Creator2/1  "F"
  Selector4/1 -> Bus Creator1/1  "F"
  Vehicle Adapter/1(VehSusp) -> Bus Selector1/1
  Bus Selector/2 -> Independent K and C Suspension/2  "<Re>"

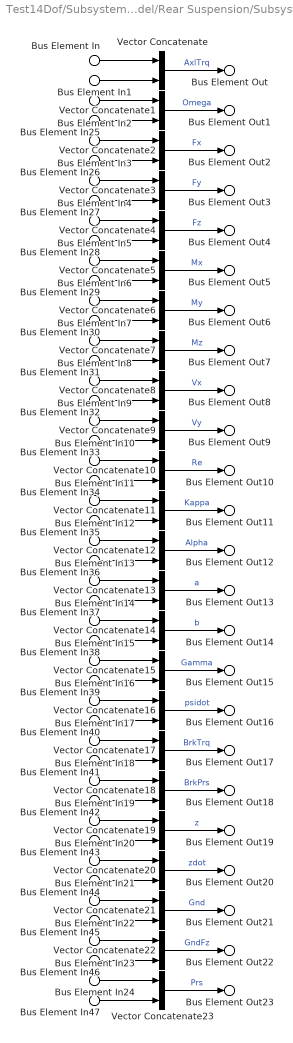
== system Test14Dof/Subsystem/Vehicle 14 DoF model/Rear Suspension/Subsystem ==
  Bus Element In : Inport  PortName=Frnt  Element=AxlTrq
  Bus Element In2 : Inport  PortName=Frnt  Element=Omega
  Bus Element In3 : Inport  PortName=Frnt  Element=Fx
  Bus Element In4 : Inport  PortName=Frnt  Element=Fy
  Bus Element In5 : Inport  PortName=Frnt  Element=Fz
  Bus Element In6 : Inport  PortName=Frnt  Element=Mx
  Bus Element In7 : Inport  PortName=Frnt  Element=My
  Bus Element In8 : Inport  PortName=Frnt  Element=Mz
  Bus Element In9 : Inport  PortName=Frnt  Element=Vx
  Bus Element In10 : Inport  PortName=Frnt  Element=Vy
  Bus Element In11 : Inport  PortName=Frnt  Element=Re
  Bus Element In12 : Inport  PortName=Frnt  Element=Kappa
  Bus Element In13 : Inport  PortName=Frnt  Element=Alpha
  Bus Element In14 : Inport  PortName=Frnt  Element=a
  Bus Element In15 : Inport  PortName=Frnt  Element=b
  Bus Element In16 : Inport  PortName=Frnt  Element=Gamma
  Bus Element In17 : Inport  PortName=Frnt  Element=psidot
  Bus Element In18 : Inport  PortName=Frnt  Element=BrkTrq
  Bus Element In19 : Inport  PortName=Frnt  Element=BrkPrs
  Bus Element In20 : Inport  PortName=Frnt  Element=z
  Bus Element In21 : Inport  PortName=Frnt  Element=zdot
  Bus Element In22 : Inport  PortName=Frnt  Element=Gnd
  Bus Element In23 : Inport  PortName=Frnt  Element=GndFz
  Bus Element In24 : Inport  PortName=Frnt  Element=Prs
  Bus Element In1 : Inport  Port=2  PortName=Rear  Element=AxlTrq
  Bus Element In25 : Inport  Port=2  PortName=Rear  Element=Omega
  Bus Element In26 : Inport  Port=2  PortName=Rear  Element=Fx
  Bus Element In27 : Inport  Port=2  PortName=Rear  Element=Fy
  Bus Element In28 : Inport  Port=2  PortName=Rear  Element=Fz
  Bus Element In29 : Inport  Port=2  PortName=Rear  Element=Mx
  Bus Element In30 : Inport  Port=2  PortName=Rear  Element=My
  Bus Element In31 : Inport  Port=2  PortName=Rear  Element=Mz
  Bus Element In32 : Inport  Port=2  PortName=Rear  Element=Vx
  Bus Element In33 : Inport  Port=2  PortName=Rear  Element=Vy
  Bus Element In34 : Inport  Port=2  PortName=Rear  Element=Re
  Bus Element In35 : Inport  Port=2  PortName=Rear  Element=Kappa
  Bus Element In36 : Inport  Port=2  PortName=Rear  Element=Alpha
  Bus Element In37 : Inport  Port=2  PortName=Rear  Element=a
  Bus Element In38 : Inport  Port=2  PortName=Rear  Element=b
  Bus Element In39 : Inport  Port=2  PortName=Rear  Element=Gamma
  Bus Element In40 : Inport  Port=2  PortName=Rear  Element=psidot
  Bus Element In41 : Inport  Port=2  PortName=Rear  Element=BrkTrq
  Bus Element In42 : Inport  Port=2  PortName=Rear  Element=BrkPrs
  Bus Element In43 : Inport  Port=2  PortName=Rear  Element=z
  Bus Element In44 : Inport  Port=2  PortName=Rear  Element=zdot
  Bus Element In45 : Inport  Port=2  PortName=Rear  Element=Gnd
  Bus Element In46 : Inport  Port=2  PortName=Rear  Element=GndFz
  Bus Element In47 : Inport  Port=2  PortName=Rear  Element=Prs
  Vector Concatenate{,1..23} (24 alike) : Concatenate
  Bus Element Out : Outport  PortName=Wheels  Element=AxlTrq
  Bus Element Out1 : Outport  PortName=Wheels  Element=Omega
  Bus Element Out2 : Outport  PortName=Wheels  Element=Fx
  Bus Element Out3 : Outport  PortName=Wheels  Element=Fy
  Bus Element Out4 : Outport  PortName=Wheels  Element=Fz
  Bus Element Out5 : Outport  PortName=Wheels  Element=Mx
  Bus Element Out6 : Outport  PortName=Wheels  Element=My
  Bus Element Out7 : Outport  PortName=Wheels  Element=Mz
  Bus Element Out8 : Outport  PortName=Wheels  Element=Vx
  Bus Element Out9 : Outport  PortName=Wheels  Element=Vy
  Bus Element Out10 : Outport  PortName=Wheels  Element=Re
  Bus Element Out11 : Outport  PortName=Wheels  Element=Kappa
  Bus Element Out12 : Outport  PortName=Wheels  Element=Alpha
  Bus Element Out13 : Outport  PortName=Wheels  Element=a
  Bus Element Out14 : Outport  PortName=Wheels  Element=b
  Bus Element Out15 : Outport  PortName=Wheels  Element=Gamma
  Bus Element Out16 : Outport  PortName=Wheels  Element=psidot
  Bus Element Out17 : Outport  PortName=Wheels  Element=BrkTrq
  Bus Element Out18 : Outport  PortName=Wheels  Element=BrkPrs
  Bus Element Out19 : Outport  PortName=Wheels  Element=z
  Bus Element Out20 : Outport  PortName=Wheels  Element=zdot
  Bus Element Out21 : Outport  PortName=Wheels  Element=Gnd
  Bus Element Out22 : Outport  PortName=Wheels  Element=GndFz
  Bus Element Out23 : Outport  PortName=Wheels  Element=Prs
  wires:
  Bus Element In/1 -> Vector Concatenate/1
  Bus Element In1/1 -> Vector Concatenate/2
  Bus Element In2/1 -> Vector Concatenate1/1
  Bus Element In25/1 -> Vector Concatenate1/2
  Bus Element In3/1 -> Vector Concatenate2/1
  Bus Element In26/1 -> Vector Concatenate2/2
  Bus Element In4/1 -> Vector Concatenate3/1
  Bus Element In27/1 -> Vector Concatenate3/2
  Bus Element In5/1 -> Vector Concatenate4/1
  Bus Element In28/1 -> Vector Concatenate4/2
  Bus Element In6/1 -> Vector Concatenate5/1
  Bus Element In29/1 -> Vector Concatenate5/2
  Bus Element In7/1 -> Vector Concatenate6/1
  Bus Element In30/1 -> Vector Concatenate6/2
  Bus Element In8/1 -> Vector Concatenate7/1
  Bus Element In31/1 -> Vector Concatenate7/2
  Bus Element In9/1 -> Vector Concatenate8/1
  Bus Element In32/1 -> Vector Concatenate8/2
  Bus Element In10/1 -> Vector Concatenate9/1
  Bus Element In33/1 -> Vector Concatenate9/2
  Bus Element In11/1 -> Vector Concatenate10/1
  Bus Element In34/1 -> Vector Concatenate10/2
  Bus Element In12/1 -> Vector Concatenate11/1
  Bus Element In35/1 -> Vector Concatenate11/2
  Bus Element In13/1 -> Vector Concatenate12/1
  Bus Element In36/1 -> Vector Concatenate12/2
  Bus Element In14/1 -> Vector Concatenate13/1
  Bus Element In37/1 -> Vector Concatenate13/2
  Bus Element In15/1 -> Vector Concatenate14/1
  Bus Element In38/1 -> Vector Concatenate14/2
  Bus Element In16/1 -> Vector Concatenate15/1
  Bus Element In39/1 -> Vector Concatenate15/2
  Bus Element In17/1 -> Vector Concatenate16/1
  Bus Element In40/1 -> Vector Concatenate16/2
  Bus Element In18/1 -> Vector Concatenate17/1
  Bus Element In41/1 -> Vector Concatenate17/2
  Bus Element In19/1 -> Vector Concatenate18/1
  Bus Element In42/1 -> Vector Concatenate18/2
  Bus Element In20/1 -> Vector Concatenate19/1
  Bus Element In43/1 -> Vector Concatenate19/2
  Bus Element In21/1 -> Vector Concatenate20/1
  Bus Element In44/1 -> Vector Concatenate20/2
  Bus Element In22/1 -> Vector Concatenate21/1
  Bus Element In45/1 -> Vector Concatenate21/2
  Bus Element In23/1 -> Vector Concatenate22/1
  Bus Element In46/1 -> Vector Concatenate22/2
  Bus Element In24/1 -> Vector Concatenate23/1
  Bus Element In47/1 -> Vector Concatenate23/2
  Vector Concatenate/1 -> Bus Element Out/1  "AxlTrq"
  Vector Concatenate1/1 -> Bus Element Out1/1  "Omega"
  Vector Concatenate2/1 -> Bus Element Out2/1  "Fx"
  Vector Concatenate3/1 -> Bus Element Out3/1  "Fy"
  Vector Concatenate4/1 -> Bus Element Out4/1  "Fz"
  Vector Concatenate5/1 -> Bus Element Out5/1  "Mx"
  Vector Concatenate6/1 -> Bus Element Out6/1  "My"
  Vector Concatenate7/1 -> Bus Element Out7/1  "Mz"
  Vector Concatenate8/1 -> Bus Element Out8/1  "Vx"
  Vector Concatenate9/1 -> Bus Element Out9/1  "Vy"
  Vector Concatenate10/1 -> Bus Element Out10/1  "Re"
  Vector Concatenate11/1 -> Bus Element Out11/1  "Kappa"
  Vector Concatenate12/1 -> Bus Element Out12/1  "Alpha"
  Vector Concatenate13/1 -> Bus Element Out13/1  "a"
  Vector Concatenate14/1 -> Bus Element Out14/1  "b"
  Vector Concatenate15/1 -> Bus Element Out15/1  "Gamma"
  Vector Concatenate16/1 -> Bus Element Out16/1  "psidot"
  Vector Concatenate17/1 -> Bus Element Out17/1  "BrkTrq"
  Vector Concatenate18/1 -> Bus Element Out18/1  "BrkPrs"
  Vector Concatenate19/1 -> Bus Element Out19/1  "z"
  Vector Concatenate20/1 -> Bus Element Out20/1  "zdot"
  Vector Concatenate21/1 -> Bus Element Out21/1  "Gnd"
  Vector Concatenate22/1 -> Bus Element Out22/1  "GndFz"
  Vector Concatenate23/1 -> Bus Element Out23/1  "Prs"

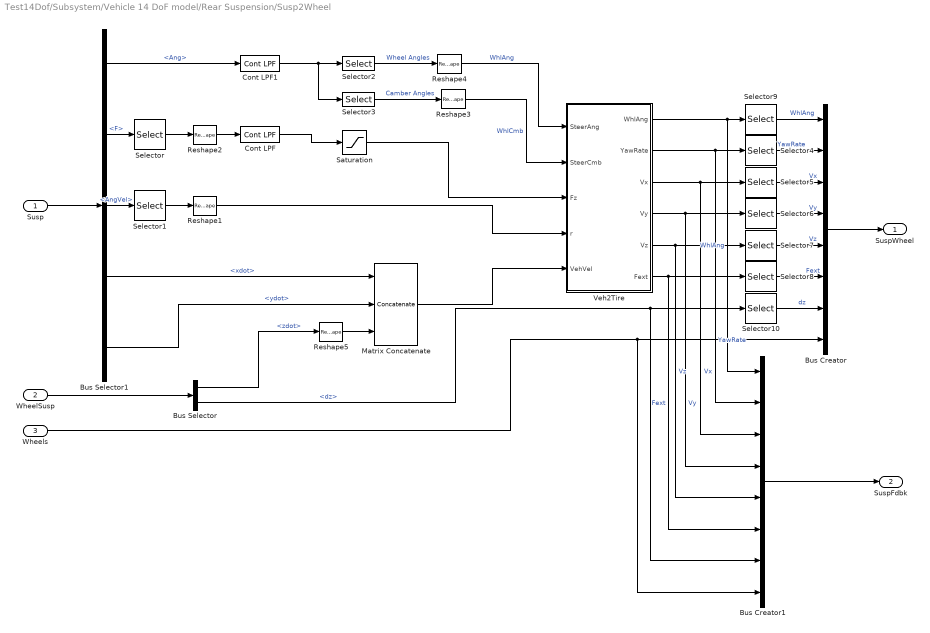
== system Test14Dof/Subsystem/Vehicle 14 DoF model/Rear Suspension/Susp2Wheel ==
  Susp : Inport
  WheelSusp : Inport  Port=2
  Wheels : Inport  Port=3
  Bus Creator : BusCreator  Inputs=8
  Bus Creator1 : BusCreator  Inputs=8
  Bus Selector : BusSelector  OutputSignals=SuspFrame.zdot,SuspFrame.dz
  Bus Selector1 : BusSelector  OutputSignals=Whl.Ang,Whl.F,Whl.AngVel,Whl.xdot,Whl.ydot
  Cont LPF : autolibutils/Cont LPF  wc=100*2*pi  AbsoluteTolerance=auto  aMode=2
  Cont LPF1 : autolibutils/Cont LPF  wc=100*2*pi  AbsoluteTolerance=auto  aMode=2
  Matrix Concatenate : Concatenate  NumInputs=3  Mode=Multidimensional array
  Reshape{1..4} (4 alike) : Reshape
  Reshape5 : Reshape  OutputDimensionality=Row vector (2-D)
  Saturation : Saturate  UpperLimit=inf  LowerLimit=-10*9.81*2000  ZeroCross=off
  Selector : Selector  NumberOfDimensions=2  InputPortWidth=3  IndexOptions=Index vector (dialog),Select all  Indices=[3],1  OutputSizes=1,1
  Selector1 : Selector  NumberOfDimensions=2  InputPortWidth=1  IndexOptions=Index vector (dialog),Select all  Indices=[3],1  OutputSizes=1,1
  Selector{4..8,10} (6 alike) : Selector  InputPortWidth=4  IndexOptions=Index vector (dialog)  Indices=[3 4]  OutputSizes=1
  Selector2 : Selector  NumberOfDimensions=2  InputPortWidth=3  IndexOptions=Index vector (dialog),Select all  Indices=3,1  OutputSizes=1,1
  Selector3 : Selector  NumberOfDimensions=2  InputPortWidth=3  IndexOptions=Index vector (dialog),Select all  Indices=1,1  OutputSizes=1,1
  Selector9 : Selector  NumberOfDimensions=2  InputPortWidth=4  IndexOptions=Index vector (dialog),Index vector (dialog)  Indices=[1 2 3],[3 4]  OutputSizes=1,1
  Veh2Tire : Subsystem
  SuspWheel : Outport
  SuspFdbk : Outport  Port=2
  wires:
  Bus Selector/2 -> Bus Creator1/7, Selector10/1  "<dz>"
  Veh2Tire/2(YawRate) -> Bus Creator1/2, Selector4/1  "YawRate"
  Bus Selector1/2 -> Selector/1  "<F>"
  Cont LPF1/1 -> Selector2/1, Selector3/1
  Reshape1/1 -> Veh2Tire/4(r)
  Selector2/1 -> Reshape4/1  "Wheel Angles"
  Reshape2/1 -> Cont LPF/1
  Selector3/1 -> Reshape3/1  "Camber Angles"
  Reshape3/1 -> Veh2Tire/2(SteerCmb)  "WhlCmb"
  Veh2Tire/1(WhlAng) -> Bus Creator1/1, Selector9/1  "WhlAng"
  Reshape4/1 -> Veh2Tire/1(SteerAng)  "WhlAng"
  Bus Selector1/4 -> Matrix Concatenate/1  "<xdot>"
  Bus Selector1/3 -> Selector1/1  "<AngVel>"
  Bus Selector1/5 -> Matrix Concatenate/2  "<ydot>"
  Veh2Tire/6(Fext) -> Bus Creator1/6, Selector8/1  "Fext"
  Selector1/1 -> Reshape1/1
  Saturation/1 -> Veh2Tire/3(Fz)
  Matrix Concatenate/1 -> Veh2Tire/5(VehVel)
  Selector/1 -> Reshape2/1
  Cont LPF/1 -> Saturation/1
  WheelSusp/1 -> Bus Selector/1
  Reshape5/1 -> Matrix Concatenate/3
  Bus Selector1/1 -> Cont LPF1/1  "<Ang>"
  Veh2Tire/5(Vz) -> Bus Creator1/5, Selector7/1  "Vz"
  Susp/1 -> Bus Selector1/1
  Veh2Tire/4(Vy) -> Bus Creator1/4, Selector6/1  "Vy"
  Veh2Tire/3(Vx) -> Bus Creator1/3, Selector5/1  "Vx"
  Bus Selector/1 -> Reshape5/1  "<zdot>"
  Bus Creator/1 -> SuspWheel/1
  Wheels/1 -> Bus Creator1/8, Bus Creator/8
  Selector4/1 -> Bus Creator/2  "YawRate"
  Selector5/1 -> Bus Creator/3  "Vx"
  Selector6/1 -> Bus Creator/4  "Vy"
  Selector7/1 -> Bus Creator/5  "Vz"
  Selector8/1 -> Bus Creator/6  "Fext"
  Selector9/1 -> Bus Creator/1  "WhlAng"
  Selector10/1 -> Bus Creator/7  "dz"
  Bus Creator1/1 -> SuspFdbk/1
